simulink model "c00005M_harness"  (R2018a)
settings: Solver=FixedStepAuto  StartTime=0.0  StopTime=300  FixedStep=0.1  RelTol=1e-3
undefined symbols (not defined in the file): A1, hmax, PriorityTank, R1, R2, sigbuilder_block, TempThreshold
(part 5 of 50)

== system c00005M_harness/M007 ==
  note: VALUES
      | ---------------------------------
      | ControlType = 1 | 2 | 3
      | FillTank = 0 | 1
      | EmptyTank = 0 | 1
      | ManualReference between 0 and 1
      | Tempreature between 0 and 100
      | EmergencyButton = 0 | 1
      | LiquidLevel between 0 and 1 (hmax)
  note: Inputs For Tank2
  note: NAMES
      | --------------------------------------------
      | CT1 = ControlType Tank 1
      | F1 = Fill Tank 1
      | E1 = Empty Tank 1
      | MR1 = Manual Reference Tank1
      | T1 = Temperature Tank 1
      | EB1 = Emergency Button Tank 1
      | LL1 = Liquid Level 1
  note: Inputs For Tank3
  note: Inputs For Tank1
  CT1 : Inport
  F1 : Inport  Port=2
  E1 : Inport  Port=3
  T1 : Inport  Port=4
  EB1 : Inport  Port=5
  CT3 : Inport  Port=6
  F3 : Inport  Port=7
  E3 : Inport  Port=8
  T3 : Inport  Port=9
  EB3 : Inport  Port=10
  Tank1 : Subsystem
  Tank3 : Subsystem
  LL1 : Outport
  LL3 : Outport  Port=2
  wires:
  EB1/1 -> Tank1/5(EB1)
  Tank3/1(LL3) -> LL3/1, Tank1/6(LL3)
  T1/1 -> Tank1/4(T1)
  Tank1/1(LL1) -> LL1/1, Tank3/6(LL1)
  E3/1 -> Tank3/3(E3)
  F1/1 -> Tank1/2(F1)
  E1/1 -> Tank1/3(E1)
  CT3/1 -> Tank3/1(CT3)
  F3/1 -> Tank3/2(F3)
  EB3/1 -> Tank3/5(EB3)
  T3/1 -> Tank3/4(T3)
  CT1/1 -> Tank1/1(CT1)

== system c00005M_harness/M008 ==
  note: VALUES
      | ---------------------------------
      | ControlType = 1 | 2 | 3
      | FillTank = 0 | 1
      | EmptyTank = 0 | 1
      | ManualReference between 0 and 1
      | Tempreature between 0 and 100
      | EmergencyButton = 0 | 1
      | LiquidLevel between 0 and 1 (hmax)
  note: Inputs For Tank2
  note: NAMES
      | --------------------------------------------
      | CT1 = ControlType Tank 1
      | F1 = Fill Tank 1
      | E1 = Empty Tank 1
      | MR1 = Manual Reference Tank1
      | T1 = Temperature Tank 1
      | EB1 = Emergency Button Tank 1
      | LL1 = Liquid Level 1
  note: Inputs For Tank3
  note: Inputs For Tank1
  CT1 : Inport
  F1 : Inport  Port=2
  E1 : Inport  Port=3
  T1 : Inport  Port=4
  EB1 : Inport  Port=5
  CT3 : Inport  Port=6
  F3 : Inport  Port=7
  E3 : Inport  Port=8
  T3 : Inport  Port=9
  EB3 : Inport  Port=10
  Tank1 : Subsystem
  Tank3 : Subsystem
  LL1 : Outport
  LL3 : Outport  Port=2
  wires:
  EB1/1 -> Tank1/5(EB1)
  Tank3/1(LL3) -> LL3/1, Tank1/6(LL3)
  T1/1 -> Tank1/4(T1)
  Tank1/1(LL1) -> LL1/1, Tank3/6(LL1)
  E3/1 -> Tank3/3(E3)
  F1/1 -> Tank1/2(F1)
  E1/1 -> Tank1/3(E1)
  CT3/1 -> Tank3/1(CT3)
  F3/1 -> Tank3/2(F3)
  EB3/1 -> Tank3/5(EB3)
  T3/1 -> Tank3/4(T3)
  CT1/1 -> Tank1/1(CT1)

== system c00005M_harness/M009 ==
  note: VALUES
      | ---------------------------------
      | ControlType = 1 | 2 | 3
      | FillTank = 0 | 1
      | EmptyTank = 0 | 1
      | ManualReference between 0 and 1
      | Tempreature between 0 and 100
      | EmergencyButton = 0 | 1
      | LiquidLevel between 0 and 1 (hmax)
  note: Inputs For Tank2
  note: NAMES
      | --------------------------------------------
      | CT1 = ControlType Tank 1
      | F1 = Fill Tank 1
      | E1 = Empty Tank 1
      | MR1 = Manual Reference Tank1
      | T1 = Temperature Tank 1
      | EB1 = Emergency Button Tank 1
      | LL1 = Liquid Level 1
  note: Inputs For Tank3
  note: Inputs For Tank1
  CT1 : Inport
  F1 : Inport  Port=2
  E1 : Inport  Port=3
  T1 : Inport  Port=4
  EB1 : Inport  Port=5
  CT3 : Inport  Port=6
  F3 : Inport  Port=7
  E3 : Inport  Port=8
  T3 : Inport  Port=9
  EB3 : Inport  Port=10
  Tank1 : Subsystem
  Tank3 : Subsystem
  LL1 : Outport
  LL3 : Outport  Port=2
  wires:
  EB1/1 -> Tank1/5(EB1)
  Tank3/1(LL3) -> LL3/1, Tank1/6(LL3)
  T1/1 -> Tank1/4(T1)
  Tank1/1(LL1) -> LL1/1, Tank3/6(LL1)
  E3/1 -> Tank3/3(E3)
  F1/1 -> Tank1/2(F1)
  E1/1 -> Tank1/3(E1)
  CT3/1 -> Tank3/1(CT3)
  F3/1 -> Tank3/2(F3)
  EB3/1 -> Tank3/5(EB3)
  T3/1 -> Tank3/4(T3)
  CT1/1 -> Tank1/1(CT1)

== system c00005M_harness/M010 ==
  note: VALUES
      | ---------------------------------
      | ControlType = 1 | 2 | 3
      | FillTank = 0 | 1
      | EmptyTank = 0 | 1
      | ManualReference between 0 and 1
      | Tempreature between 0 and 100
      | EmergencyButton = 0 | 1
      | LiquidLevel between 0 and 1 (hmax)
  note: Inputs For Tank2
  note: NAMES
      | --------------------------------------------
      | CT1 = ControlType Tank 1
      | F1 = Fill Tank 1
      | E1 = Empty Tank 1
      | MR1 = Manual Reference Tank1
      | T1 = Temperature Tank 1
      | EB1 = Emergency Button Tank 1
      | LL1 = Liquid Level 1
  note: Inputs For Tank3
  note: Inputs For Tank1
  CT1 : Inport
  F1 : Inport  Port=2
  E1 : Inport  Port=3
  T1 : Inport  Port=4
  EB1 : Inport  Port=5
  CT3 : Inport  Port=6
  F3 : Inport  Port=7
  E3 : Inport  Port=8
  T3 : Inport  Port=9
  EB3 : Inport  Port=10
  Tank1 : Subsystem
  Tank3 : Subsystem
  LL1 : Outport
  LL3 : Outport  Port=2
  wires:
  EB1/1 -> Tank1/5(EB1)
  Tank3/1(LL3) -> LL3/1, Tank1/6(LL3)
  T1/1 -> Tank1/4(T1)
  Tank1/1(LL1) -> LL1/1, Tank3/6(LL1)
  E3/1 -> Tank3/3(E3)
  F1/1 -> Tank1/2(F1)
  E1/1 -> Tank1/3(E1)
  CT3/1 -> Tank3/1(CT3)
  F3/1 -> Tank3/2(F3)
  EB3/1 -> Tank3/5(EB3)
  T3/1 -> Tank3/4(T3)
  CT1/1 -> Tank1/1(CT1)

== system c00005M_harness/M011 ==
  note: VALUES
      | ---------------------------------
      | ControlType = 1 | 2 | 3
      | FillTank = 0 | 1
      | EmptyTank = 0 | 1
      | ManualReference between 0 and 1
      | Tempreature between 0 and 100
      | EmergencyButton = 0 | 1
      | LiquidLevel between 0 and 1 (hmax)
  note: Inputs For Tank2
  note: NAMES
      | --------------------------------------------
      | CT1 = ControlType Tank 1
      | F1 = Fill Tank 1
      | E1 = Empty Tank 1
      | MR1 = Manual Reference Tank1
      | T1 = Temperature Tank 1
      | EB1 = Emergency Button Tank 1
      | LL1 = Liquid Level 1
  note: Inputs For Tank3
  note: Inputs For Tank1
  CT1 : Inport
  F1 : Inport  Port=2
  E1 : Inport  Port=3
  T1 : Inport  Port=4
  EB1 : Inport  Port=5
  CT3 : Inport  Port=6
  F3 : Inport  Port=7
  E3 : Inport  Port=8
  T3 : Inport  Port=9
  EB3 : Inport  Port=10
  Tank1 : Subsystem
  Tank3 : Subsystem
  LL1 : Outport
  LL3 : Outport  Port=2
  wires:
  EB1/1 -> Tank1/5(EB1)
  Tank3/1(LL3) -> LL3/1, Tank1/6(LL3)
  T1/1 -> Tank1/4(T1)
  Tank1/1(LL1) -> LL1/1, Tank3/6(LL1)
  E3/1 -> Tank3/3(E3)
  F1/1 -> Tank1/2(F1)
  E1/1 -> Tank1/3(E1)
  CT3/1 -> Tank3/1(CT3)
  F3/1 -> Tank3/2(F3)
  EB3/1 -> Tank3/5(EB3)
  T3/1 -> Tank3/4(T3)
  CT1/1 -> Tank1/1(CT1)

== system c00005M_harness/M012 ==
  note: VALUES
      | ---------------------------------
      | ControlType = 1 | 2 | 3
      | FillTank = 0 | 1
      | EmptyTank = 0 | 1
      | ManualReference between 0 and 1
      | Tempreature between 0 and 100
      | EmergencyButton = 0 | 1
      | LiquidLevel between 0 and 1 (hmax)
  note: Inputs For Tank2
  note: NAMES
      | --------------------------------------------
      | CT1 = ControlType Tank 1
      | F1 = Fill Tank 1
      | E1 = Empty Tank 1
      | MR1 = Manual Reference Tank1
      | T1 = Temperature Tank 1
      | EB1 = Emergency Button Tank 1
      | LL1 = Liquid Level 1
  note: Inputs For Tank3
  note: Inputs For Tank1
  CT1 : Inport
  F1 : Inport  Port=2
  E1 : Inport  Port=3
  T1 : Inport  Port=4
  EB1 : Inport  Port=5
  CT3 : Inport  Port=6
  F3 : Inport  Port=7
  E3 : Inport  Port=8
  T3 : Inport  Port=9
  EB3 : Inport  Port=10
  Tank1 : Subsystem
  Tank3 : Subsystem
  LL1 : Outport
  LL3 : Outport  Port=2
  wires:
  EB1/1 -> Tank1/5(EB1)
  Tank3/1(LL3) -> LL3/1, Tank1/6(LL3)
  T1/1 -> Tank1/4(T1)
  Tank1/1(LL1) -> LL1/1, Tank3/6(LL1)
  E3/1 -> Tank3/3(E3)
  F1/1 -> Tank1/2(F1)
  E1/1 -> Tank1/3(E1)
  CT3/1 -> Tank3/1(CT3)
  F3/1 -> Tank3/2(F3)
  EB3/1 -> Tank3/5(EB3)
  T3/1 -> Tank3/4(T3)
  CT1/1 -> Tank1/1(CT1)

== system c00005M_harness/M013 ==
  note: VALUES
      | ---------------------------------
      | ControlType = 1 | 2 | 3
      | FillTank = 0 | 1
      | EmptyTank = 0 | 1
      | ManualReference between 0 and 1
      | Tempreature between 0 and 100
      | EmergencyButton = 0 | 1
      | LiquidLevel between 0 and 1 (hmax)
  note: Inputs For Tank2
  note: NAMES
      | --------------------------------------------
      | CT1 = ControlType Tank 1
      | F1 = Fill Tank 1
      | E1 = Empty Tank 1
      | MR1 = Manual Reference Tank1
      | T1 = Temperature Tank 1
      | EB1 = Emergency Button Tank 1
      | LL1 = Liquid Level 1
  note: Inputs For Tank3
  note: Inputs For Tank1
  CT1 : Inport
  F1 : Inport  Port=2
  E1 : Inport  Port=3
  T1 : Inport  Port=4
  EB1 : Inport  Port=5
  CT3 : Inport  Port=6
  F3 : Inport  Port=7
  E3 : Inport  Port=8
  T3 : Inport  Port=9
  EB3 : Inport  Port=10
  Tank1 : Subsystem
  Tank3 : Subsystem
  LL1 : Outport
  LL3 : Outport  Port=2
  wires:
  EB1/1 -> Tank1/5(EB1)
  Tank3/1(LL3) -> LL3/1, Tank1/6(LL3)
  T1/1 -> Tank1/4(T1)
  Tank1/1(LL1) -> LL1/1, Tank3/6(LL1)
  E3/1 -> Tank3/3(E3)
  F1/1 -> Tank1/2(F1)
  E1/1 -> Tank1/3(E1)
  CT3/1 -> Tank3/1(CT3)
  F3/1 -> Tank3/2(F3)
  EB3/1 -> Tank3/5(EB3)
  T3/1 -> Tank3/4(T3)
  CT1/1 -> Tank1/1(CT1)

== system c00005M_harness/M014 ==
  note: VALUES
      | ---------------------------------
      | ControlType = 1 | 2 | 3
      | FillTank = 0 | 1
      | EmptyTank = 0 | 1
      | ManualReference between 0 and 1
      | Tempreature between 0 and 100
      | EmergencyButton = 0 | 1
      | LiquidLevel between 0 and 1 (hmax)
  note: Inputs For Tank2
  note: NAMES
      | --------------------------------------------
      | CT1 = ControlType Tank 1
      | F1 = Fill Tank 1
      | E1 = Empty Tank 1
      | MR1 = Manual Reference Tank1
      | T1 = Temperature Tank 1
      | EB1 = Emergency Button Tank 1
      | LL1 = Liquid Level 1
  note: Inputs For Tank3
  note: Inputs For Tank1
  CT1 : Inport
  F1 : Inport  Port=2
  E1 : Inport  Port=3
  T1 : Inport  Port=4
  EB1 : Inport  Port=5
  CT3 : Inport  Port=6
  F3 : Inport  Port=7
  E3 : Inport  Port=8
  T3 : Inport  Port=9
  EB3 : Inport  Port=10
  Tank1 : Subsystem
  Tank3 : Subsystem
  LL1 : Outport
  LL3 : Outport  Port=2
  wires:
  EB1/1 -> Tank1/5(EB1)
  Tank3/1(LL3) -> LL3/1, Tank1/6(LL3)
  T1/1 -> Tank1/4(T1)
  Tank1/1(LL1) -> LL1/1, Tank3/6(LL1)
  E3/1 -> Tank3/3(E3)
  F1/1 -> Tank1/2(F1)
  E1/1 -> Tank1/3(E1)
  CT3/1 -> Tank3/1(CT3)
  F3/1 -> Tank3/2(F3)
  EB3/1 -> Tank3/5(EB3)
  T3/1 -> Tank3/4(T3)
  CT1/1 -> Tank1/1(CT1)

== system c00005M_harness/M015 ==
  note: VALUES
      | ---------------------------------
      | ControlType = 1 | 2 | 3
      | FillTank = 0 | 1
      | EmptyTank = 0 | 1
      | ManualReference between 0 and 1
      | Tempreature between 0 and 100
      | EmergencyButton = 0 | 1
      | LiquidLevel between 0 and 1 (hmax)
  note: Inputs For Tank2
  note: NAMES
      | --------------------------------------------
      | CT1 = ControlType Tank 1
      | F1 = Fill Tank 1
      | E1 = Empty Tank 1
      | MR1 = Manual Reference Tank1
      | T1 = Temperature Tank 1
      | EB1 = Emergency Button Tank 1
      | LL1 = Liquid Level 1
  note: Inputs For Tank3
  note: Inputs For Tank1
  CT1 : Inport
  F1 : Inport  Port=2
  E1 : Inport  Port=3
  T1 : Inport  Port=4
  EB1 : Inport  Port=5
  CT3 : Inport  Port=6
  F3 : Inport  Port=7
  E3 : Inport  Port=8
  T3 : Inport  Port=9
  EB3 : Inport  Port=10
  Tank1 : Subsystem
  Tank3 : Subsystem
  LL1 : Outport
  LL3 : Outport  Port=2
  wires:
  EB1/1 -> Tank1/5(EB1)
  Tank3/1(LL3) -> LL3/1, Tank1/6(LL3)
  T1/1 -> Tank1/4(T1)
  Tank1/1(LL1) -> LL1/1, Tank3/6(LL1)
  E3/1 -> Tank3/3(E3)
  F1/1 -> Tank1/2(F1)
  E1/1 -> Tank1/3(E1)
  CT3/1 -> Tank3/1(CT3)
  F3/1 -> Tank3/2(F3)
  EB3/1 -> Tank3/5(EB3)
  T3/1 -> Tank3/4(T3)
  CT1/1 -> Tank1/1(CT1)

== system c00005M_harness/M016 ==
  note: VALUES
      | ---------------------------------
      | ControlType = 1 | 2 | 3
      | FillTank = 0 | 1
      | EmptyTank = 0 | 1
      | ManualReference between 0 and 1
      | Tempreature between 0 and 100
      | EmergencyButton = 0 | 1
      | LiquidLevel between 0 and 1 (hmax)
  note: Inputs For Tank2
  note: NAMES
      | --------------------------------------------
      | CT1 = ControlType Tank 1
      | F1 = Fill Tank 1
      | E1 = Empty Tank 1
      | MR1 = Manual Reference Tank1
      | T1 = Temperature Tank 1
      | EB1 = Emergency Button Tank 1
      | LL1 = Liquid Level 1
  note: Inputs For Tank3
  note: Inputs For Tank1
  CT1 : Inport
  F1 : Inport  Port=2
  E1 : Inport  Port=3
  T1 : Inport  Port=4
  EB1 : Inport  Port=5
  CT3 : Inport  Port=6
  F3 : Inport  Port=7
  E3 : Inport  Port=8
  T3 : Inport  Port=9
  EB3 : Inport  Port=10
  Tank1 : Subsystem
  Tank3 : Subsystem
  LL1 : Outport
  LL3 : Outport  Port=2
  wires:
  EB1/1 -> Tank1/5(EB1)
  Tank3/1(LL3) -> LL3/1, Tank1/6(LL3)
  T1/1 -> Tank1/4(T1)
  Tank1/1(LL1) -> LL1/1, Tank3/6(LL1)
  E3/1 -> Tank3/3(E3)
  F1/1 -> Tank1/2(F1)
  E1/1 -> Tank1/3(E1)
  CT3/1 -> Tank3/1(CT3)
  F3/1 -> Tank3/2(F3)
  EB3/1 -> Tank3/5(EB3)
  T3/1 -> Tank3/4(T3)
  CT1/1 -> Tank1/1(CT1)

== system c00005M_harness/M017 ==
  note: VALUES
      | ---------------------------------
      | ControlType = 1 | 2 | 3
      | FillTank = 0 | 1
      | EmptyTank = 0 | 1
      | ManualReference between 0 and 1
      | Tempreature between 0 and 100
      | EmergencyButton = 0 | 1
      | LiquidLevel between 0 and 1 (hmax)
  note: Inputs For Tank2
  note: NAMES
      | --------------------------------------------
      | CT1 = ControlType Tank 1
      | F1 = Fill Tank 1
      | E1 = Empty Tank 1
      | MR1 = Manual Reference Tank1
      | T1 = Temperature Tank 1
      | EB1 = Emergency Button Tank 1
      | LL1 = Liquid Level 1
  note: Inputs For Tank3
  note: Inputs For Tank1
  CT1 : Inport
  F1 : Inport  Port=2
  E1 : Inport  Port=3
  T1 : Inport  Port=4
  EB1 : Inport  Port=5
  CT3 : Inport  Port=6
  F3 : Inport  Port=7
  E3 : Inport  Port=8
  T3 : Inport  Port=9
  EB3 : Inport  Port=10
  Tank1 : Subsystem
  Tank3 : Subsystem
  LL1 : Outport
  LL3 : Outport  Port=2
  wires:
  EB1/1 -> Tank1/5(EB1)
  Tank3/1(LL3) -> LL3/1, Tank1/6(LL3)
  T1/1 -> Tank1/4(T1)
  Tank1/1(LL1) -> LL1/1, Tank3/6(LL1)
  E3/1 -> Tank3/3(E3)
  F1/1 -> Tank1/2(F1)
  E1/1 -> Tank1/3(E1)
  CT3/1 -> Tank3/1(CT3)
  F3/1 -> Tank3/2(F3)
  EB3/1 -> Tank3/5(EB3)
  T3/1 -> Tank3/4(T3)
  CT1/1 -> Tank1/1(CT1)

== system c00005M_harness/M018 ==
  note: VALUES
      | ---------------------------------
      | ControlType = 1 | 2 | 3
      | FillTank = 0 | 1
      | EmptyTank = 0 | 1
      | ManualReference between 0 and 1
      | Tempreature between 0 and 100
      | EmergencyButton = 0 | 1
      | LiquidLevel between 0 and 1 (hmax)
  note: Inputs For Tank2
  note: NAMES
      | --------------------------------------------
      | CT1 = ControlType Tank 1
      | F1 = Fill Tank 1
      | E1 = Empty Tank 1
      | MR1 = Manual Reference Tank1
      | T1 = Temperature Tank 1
      | EB1 = Emergency Button Tank 1
      | LL1 = Liquid Level 1
  note: Inputs For Tank3
  note: Inputs For Tank1
  CT1 : Inport
  F1 : Inport  Port=2
  E1 : Inport  Port=3
  T1 : Inport  Port=4
  EB1 : Inport  Port=5
  CT3 : Inport  Port=6
  F3 : Inport  Port=7
  E3 : Inport  Port=8
  T3 : Inport  Port=9
  EB3 : Inport  Port=10
  Tank1 : Subsystem
  Tank3 : Subsystem
  LL1 : Outport
  LL3 : Outport  Port=2
  wires:
  EB1/1 -> Tank1/5(EB1)
  Tank3/1(LL3) -> LL3/1, Tank1/6(LL3)
  T1/1 -> Tank1/4(T1)
  Tank1/1(LL1) -> LL1/1, Tank3/6(LL1)
  E3/1 -> Tank3/3(E3)
  F1/1 -> Tank1/2(F1)
  E1/1 -> Tank1/3(E1)
  CT3/1 -> Tank3/1(CT3)
  F3/1 -> Tank3/2(F3)
  EB3/1 -> Tank3/5(EB3)
  T3/1 -> Tank3/4(T3)
  CT1/1 -> Tank1/1(CT1)

== system c00005M_harness/M019 ==
  note: VALUES
      | ---------------------------------
      | ControlType = 1 | 2 | 3
      | FillTank = 0 | 1
      | EmptyTank = 0 | 1
      | ManualReference between 0 and 1
      | Tempreature between 0 and 100
      | EmergencyButton = 0 | 1
      | LiquidLevel between 0 and 1 (hmax)
  note: Inputs For Tank2
  note: NAMES
      | --------------------------------------------
      | CT1 = ControlType Tank 1
      | F1 = Fill Tank 1
      | E1 = Empty Tank 1
      | MR1 = Manual Reference Tank1
      | T1 = Temperature Tank 1
      | EB1 = Emergency Button Tank 1
      | LL1 = Liquid Level 1
  note: Inputs For Tank3
  note: Inputs For Tank1
  CT1 : Inport
  F1 : Inport  Port=2
  E1 : Inport  Port=3
  T1 : Inport  Port=4
  EB1 : Inport  Port=5
  CT3 : Inport  Port=6
  F3 : Inport  Port=7
  E3 : Inport  Port=8
  T3 : Inport  Port=9
  EB3 : Inport  Port=10
  Tank1 : Subsystem
  Tank3 : Subsystem
  LL1 : Outport
  LL3 : Outport  Port=2
  wires:
  EB1/1 -> Tank1/5(EB1)
  Tank3/1(LL3) -> LL3/1, Tank1/6(LL3)
  T1/1 -> Tank1/4(T1)
  Tank1/1(LL1) -> LL1/1, Tank3/6(LL1)
  E3/1 -> Tank3/3(E3)
  F1/1 -> Tank1/2(F1)
  E1/1 -> Tank1/3(E1)
  CT3/1 -> Tank3/1(CT3)
  F3/1 -> Tank3/2(F3)
  EB3/1 -> Tank3/5(EB3)
  T3/1 -> Tank3/4(T3)
  CT1/1 -> Tank1/1(CT1)

== system c00005M_harness/M020 ==
  note: VALUES
      | ---------------------------------
      | ControlType = 1 | 2 | 3
      | FillTank = 0 | 1
      | EmptyTank = 0 | 1
      | ManualReference between 0 and 1
      | Tempreature between 0 and 100
      | EmergencyButton = 0 | 1
      | LiquidLevel between 0 and 1 (hmax)
  note: Inputs For Tank2
  note: NAMES
      | --------------------------------------------
      | CT1 = ControlType Tank 1
      | F1 = Fill Tank 1
      | E1 = Empty Tank 1
      | MR1 = Manual Reference Tank1
      | T1 = Temperature Tank 1
      | EB1 = Emergency Button Tank 1
      | LL1 = Liquid Level 1
  note: Inputs For Tank3
  note: Inputs For Tank1
  CT1 : Inport
  F1 : Inport  Port=2
  E1 : Inport  Port=3
  T1 : Inport  Port=4
  EB1 : Inport  Port=5
  CT3 : Inport  Port=6
  F3 : Inport  Port=7
  E3 : Inport  Port=8
  T3 : Inport  Port=9
  EB3 : Inport  Port=10
  Tank1 : Subsystem
  Tank3 : Subsystem
  LL1 : Outport
  LL3 : Outport  Port=2
  wires:
  EB1/1 -> Tank1/5(EB1)
  Tank3/1(LL3) -> LL3/1, Tank1/6(LL3)
  T1/1 -> Tank1/4(T1)
  Tank1/1(LL1) -> LL1/1, Tank3/6(LL1)
  E3/1 -> Tank3/3(E3)
  F1/1 -> Tank1/2(F1)
  E1/1 -> Tank1/3(E1)
  CT3/1 -> Tank3/1(CT3)
  F3/1 -> Tank3/2(F3)
  EB3/1 -> Tank3/5(EB3)
  T3/1 -> Tank3/4(T3)
  CT1/1 -> Tank1/1(CT1)

== system c00005M_harness/M021 ==
  note: VALUES
      | ---------------------------------
      | ControlType = 1 | 2 | 3
      | FillTank = 0 | 1
      | EmptyTank = 0 | 1
      | ManualReference between 0 and 1
      | Tempreature between 0 and 100
      | EmergencyButton = 0 | 1
      | LiquidLevel between 0 and 1 (hmax)
  note: Inputs For Tank2
  note: NAMES
      | --------------------------------------------
      | CT1 = ControlType Tank 1
      | F1 = Fill Tank 1
      | E1 = Empty Tank 1
      | MR1 = Manual Reference Tank1
      | T1 = Temperature Tank 1
      | EB1 = Emergency Button Tank 1
      | LL1 = Liquid Level 1
  note: Inputs For Tank3
  note: Inputs For Tank1
  CT1 : Inport
  F1 : Inport  Port=2
  E1 : Inport  Port=3
  T1 : Inport  Port=4
  EB1 : Inport  Port=5
  CT3 : Inport  Port=6
  F3 : Inport  Port=7
  E3 : Inport  Port=8
  T3 : Inport  Port=9
  EB3 : Inport  Port=10
  Tank1 : Subsystem
  Tank3 : Subsystem
  LL1 : Outport
  LL3 : Outport  Port=2
  wires:
  EB1/1 -> Tank1/5(EB1)
  Tank3/1(LL3) -> LL3/1, Tank1/6(LL3)
  T1/1 -> Tank1/4(T1)
  Tank1/1(LL1) -> LL1/1, Tank3/6(LL1)
  E3/1 -> Tank3/3(E3)
  F1/1 -> Tank1/2(F1)
  E1/1 -> Tank1/3(E1)
  CT3/1 -> Tank3/1(CT3)
  F3/1 -> Tank3/2(F3)
  EB3/1 -> Tank3/5(EB3)
  T3/1 -> Tank3/4(T3)
  CT1/1 -> Tank1/1(CT1)

== system c00005M_harness/M022 ==
  note: VALUES
      | ---------------------------------
      | ControlType = 1 | 2 | 3
      | FillTank = 0 | 1
      | EmptyTank = 0 | 1
      | ManualReference between 0 and 1
      | Tempreature between 0 and 100
      | EmergencyButton = 0 | 1
      | LiquidLevel between 0 and 1 (hmax)
  note: Inputs For Tank2
  note: NAMES
      | --------------------------------------------
      | CT1 = ControlType Tank 1
      | F1 = Fill Tank 1
      | E1 = Empty Tank 1
      | MR1 = Manual Reference Tank1
      | T1 = Temperature Tank 1
      | EB1 = Emergency Button Tank 1
      | LL1 = Liquid Level 1
  note: Inputs For Tank3
  note: Inputs For Tank1
  CT1 : Inport
  F1 : Inport  Port=2
  E1 : Inport  Port=3
  T1 : Inport  Port=4
  EB1 : Inport  Port=5
  CT3 : Inport  Port=6
  F3 : Inport  Port=7
  E3 : Inport  Port=8
  T3 : Inport  Port=9
  EB3 : Inport  Port=10
  Tank1 : Subsystem
  Tank3 : Subsystem
  LL1 : Outport
  LL3 : Outport  Port=2
  wires:
  EB1/1 -> Tank1/5(EB1)
  Tank3/1(LL3) -> LL3/1, Tank1/6(LL3)
  T1/1 -> Tank1/4(T1)
  Tank1/1(LL1) -> LL1/1, Tank3/6(LL1)
  E3/1 -> Tank3/3(E3)
  F1/1 -> Tank1/2(F1)
  E1/1 -> Tank1/3(E1)
  CT3/1 -> Tank3/1(CT3)
  F3/1 -> Tank3/2(F3)
  EB3/1 -> Tank3/5(EB3)
  T3/1 -> Tank3/4(T3)
  CT1/1 -> Tank1/1(CT1)

== system c00005M_harness/M023 ==
  note: VALUES
      | ---------------------------------
      | ControlType = 1 | 2 | 3
      | FillTank = 0 | 1
      | EmptyTank = 0 | 1
      | ManualReference between 0 and 1
      | Tempreature between 0 and 100
      | EmergencyButton = 0 | 1
      | LiquidLevel between 0 and 1 (hmax)
  note: Inputs For Tank2
  note: NAMES
      | --------------------------------------------
      | CT1 = ControlType Tank 1
      | F1 = Fill Tank 1
      | E1 = Empty Tank 1
      | MR1 = Manual Reference Tank1
      | T1 = Temperature Tank 1
      | EB1 = Emergency Button Tank 1
      | LL1 = Liquid Level 1
  note: Inputs For Tank3
  note: Inputs For Tank1
  CT1 : Inport
  F1 : Inport  Port=2
  E1 : Inport  Port=3
  T1 : Inport  Port=4
  EB1 : Inport  Port=5
  CT3 : Inport  Port=6
  F3 : Inport  Port=7
  E3 : Inport  Port=8
  T3 : Inport  Port=9
  EB3 : Inport  Port=10
  Tank1 : Subsystem
  Tank3 : Subsystem
  LL1 : Outport
  LL3 : Outport  Port=2
  wires:
  EB1/1 -> Tank1/5(EB1)
  Tank3/1(LL3) -> LL3/1, Tank1/6(LL3)
  T1/1 -> Tank1/4(T1)
  Tank1/1(LL1) -> LL1/1, Tank3/6(LL1)
  E3/1 -> Tank3/3(E3)
  F1/1 -> Tank1/2(F1)
  E1/1 -> Tank1/3(E1)
  CT3/1 -> Tank3/1(CT3)
  F3/1 -> Tank3/2(F3)
  EB3/1 -> Tank3/5(EB3)
  T3/1 -> Tank3/4(T3)
  CT1/1 -> Tank1/1(CT1)

== system c00005M_harness/M024 ==
  note: VALUES
      | ---------------------------------
      | ControlType = 1 | 2 | 3
      | FillTank = 0 | 1
      | EmptyTank = 0 | 1
      | ManualReference between 0 and 1
      | Tempreature between 0 and 100
      | EmergencyButton = 0 | 1
      | LiquidLevel between 0 and 1 (hmax)
  note: Inputs For Tank2
  note: NAMES
      | --------------------------------------------
      | CT1 = ControlType Tank 1
      | F1 = Fill Tank 1
      | E1 = Empty Tank 1
      | MR1 = Manual Reference Tank1
      | T1 = Temperature Tank 1
      | EB1 = Emergency Button Tank 1
      | LL1 = Liquid Level 1
  note: Inputs For Tank3
  note: Inputs For Tank1
  CT1 : Inport
  F1 : Inport  Port=2
  E1 : Inport  Port=3
  T1 : Inport  Port=4
  EB1 : Inport  Port=5
  CT3 : Inport  Port=6
  F3 : Inport  Port=7
  E3 : Inport  Port=8
  T3 : Inport  Port=9
  EB3 : Inport  Port=10
  Tank1 : Subsystem
  Tank3 : Subsystem
  LL1 : Outport
  LL3 : Outport  Port=2
  wires:
  EB1/1 -> Tank1/5(EB1)
  Tank3/1(LL3) -> LL3/1, Tank1/6(LL3)
  T1/1 -> Tank1/4(T1)
  Tank1/1(LL1) -> LL1/1, Tank3/6(LL1)
  E3/1 -> Tank3/3(E3)
  F1/1 -> Tank1/2(F1)
  E1/1 -> Tank1/3(E1)
  CT3/1 -> Tank3/1(CT3)
  F3/1 -> Tank3/2(F3)
  EB3/1 -> Tank3/5(EB3)
  T3/1 -> Tank3/4(T3)
  CT1/1 -> Tank1/1(CT1)

== system c00005M_harness/M025 ==
  note: VALUES
      | ---------------------------------
      | ControlType = 1 | 2 | 3
      | FillTank = 0 | 1
      | EmptyTank = 0 | 1
      | ManualReference between 0 and 1
      | Tempreature between 0 and 100
      | EmergencyButton = 0 | 1
      | LiquidLevel between 0 and 1 (hmax)
  note: Inputs For Tank2
  note: NAMES
      | --------------------------------------------
      | CT1 = ControlType Tank 1
      | F1 = Fill Tank 1
      | E1 = Empty Tank 1
      | MR1 = Manual Reference Tank1
      | T1 = Temperature Tank 1
      | EB1 = Emergency Button Tank 1
      | LL1 = Liquid Level 1
  note: Inputs For Tank3
  note: Inputs For Tank1
  CT1 : Inport
  F1 : Inport  Port=2
  E1 : Inport  Port=3
  T1 : Inport  Port=4
  EB1 : Inport  Port=5
  CT3 : Inport  Port=6
  F3 : Inport  Port=7
  E3 : Inport  Port=8
  T3 : Inport  Port=9
  EB3 : Inport  Port=10
  Tank1 : Subsystem
  Tank3 : Subsystem
  LL1 : Outport
  LL3 : Outport  Port=2
  wires:
  EB1/1 -> Tank1/5(EB1)
  Tank3/1(LL3) -> LL3/1, Tank1/6(LL3)
  T1/1 -> Tank1/4(T1)
  Tank1/1(LL1) -> LL1/1, Tank3/6(LL1)
  E3/1 -> Tank3/3(E3)
  F1/1 -> Tank1/2(F1)
  E1/1 -> Tank1/3(E1)
  CT3/1 -> Tank3/1(CT3)
  F3/1 -> Tank3/2(F3)
  EB3/1 -> Tank3/5(EB3)
  T3/1 -> Tank3/4(T3)
  CT1/1 -> Tank1/1(CT1)

== system c00005M_harness/M026 ==
  note: VALUES
      | ---------------------------------
      | ControlType = 1 | 2 | 3
      | FillTank = 0 | 1
      | EmptyTank = 0 | 1
      | ManualReference between 0 and 1
      | Tempreature between 0 and 100
      | EmergencyButton = 0 | 1
      | LiquidLevel between 0 and 1 (hmax)
  note: Inputs For Tank2
  note: NAMES
      | --------------------------------------------
      | CT1 = ControlType Tank 1
      | F1 = Fill Tank 1
      | E1 = Empty Tank 1
      | MR1 = Manual Reference Tank1
      | T1 = Temperature Tank 1
      | EB1 = Emergency Button Tank 1
      | LL1 = Liquid Level 1
  note: Inputs For Tank3
  note: Inputs For Tank1
  CT1 : Inport
  F1 : Inport  Port=2
  E1 : Inport  Port=3
  T1 : Inport  Port=4
  EB1 : Inport  Port=5
  CT3 : Inport  Port=6
  F3 : Inport  Port=7
  E3 : Inport  Port=8
  T3 : Inport  Port=9
  EB3 : Inport  Port=10
  Tank1 : Subsystem
  Tank3 : Subsystem
  LL1 : Outport
  LL3 : Outport  Port=2
  wires:
  EB1/1 -> Tank1/5(EB1)
  Tank3/1(LL3) -> LL3/1, Tank1/6(LL3)
  T1/1 -> Tank1/4(T1)
  Tank1/1(LL1) -> LL1/1, Tank3/6(LL1)
  E3/1 -> Tank3/3(E3)
  F1/1 -> Tank1/2(F1)
  E1/1 -> Tank1/3(E1)
  CT3/1 -> Tank3/1(CT3)
  F3/1 -> Tank3/2(F3)
  EB3/1 -> Tank3/5(EB3)
  T3/1 -> Tank3/4(T3)
  CT1/1 -> Tank1/1(CT1)

== system c00005M_harness/M027 ==
  note: VALUES
      | ---------------------------------
      | ControlType = 1 | 2 | 3
      | FillTank = 0 | 1
      | EmptyTank = 0 | 1
      | ManualReference between 0 and 1
      | Tempreature between 0 and 100
      | EmergencyButton = 0 | 1
      | LiquidLevel between 0 and 1 (hmax)
  note: Inputs For Tank2
  note: NAMES
      | --------------------------------------------
      | CT1 = ControlType Tank 1
      | F1 = Fill Tank 1
      | E1 = Empty Tank 1
      | MR1 = Manual Reference Tank1
      | T1 = Temperature Tank 1
      | EB1 = Emergency Button Tank 1
      | LL1 = Liquid Level 1
  note: Inputs For Tank3
  note: Inputs For Tank1
  CT1 : Inport
  F1 : Inport  Port=2
  E1 : Inport  Port=3
  T1 : Inport  Port=4
  EB1 : Inport  Port=5
  CT3 : Inport  Port=6
  F3 : Inport  Port=7
  E3 : Inport  Port=8
  T3 : Inport  Port=9
  EB3 : Inport  Port=10
  Tank1 : Subsystem
  Tank3 : Subsystem
  LL1 : Outport
  LL3 : Outport  Port=2
  wires:
  EB1/1 -> Tank1/5(EB1)
  Tank3/1(LL3) -> LL3/1, Tank1/6(LL3)
  T1/1 -> Tank1/4(T1)
  Tank1/1(LL1) -> LL1/1, Tank3/6(LL1)
  E3/1 -> Tank3/3(E3)
  F1/1 -> Tank1/2(F1)
  E1/1 -> Tank1/3(E1)
  CT3/1 -> Tank3/1(CT3)
  F3/1 -> Tank3/2(F3)
  EB3/1 -> Tank3/5(EB3)
  T3/1 -> Tank3/4(T3)
  CT1/1 -> Tank1/1(CT1)

== system c00005M_harness/M028 ==
  note: VALUES
      | ---------------------------------
      | ControlType = 1 | 2 | 3
      | FillTank = 0 | 1
      | EmptyTank = 0 | 1
      | ManualReference between 0 and 1
      | Tempreature between 0 and 100
      | EmergencyButton = 0 | 1
      | LiquidLevel between 0 and 1 (hmax)
  note: Inputs For Tank2
  note: NAMES
      | --------------------------------------------
      | CT1 = ControlType Tank 1
      | F1 = Fill Tank 1
      | E1 = Empty Tank 1
      | MR1 = Manual Reference Tank1
      | T1 = Temperature Tank 1
      | EB1 = Emergency Button Tank 1
      | LL1 = Liquid Level 1
  note: Inputs For Tank3
  note: Inputs For Tank1
  CT1 : Inport
  F1 : Inport  Port=2
  E1 : Inport  Port=3
  T1 : Inport  Port=4
  EB1 : Inport  Port=5
  CT3 : Inport  Port=6
  F3 : Inport  Port=7
  E3 : Inport  Port=8
  T3 : Inport  Port=9
  EB3 : Inport  Port=10
  Tank1 : Subsystem
  Tank3 : Subsystem
  LL1 : Outport
  LL3 : Outport  Port=2
  wires:
  EB1/1 -> Tank1/5(EB1)
  Tank3/1(LL3) -> LL3/1, Tank1/6(LL3)
  T1/1 -> Tank1/4(T1)
  Tank1/1(LL1) -> LL1/1, Tank3/6(LL1)
  E3/1 -> Tank3/3(E3)
  F1/1 -> Tank1/2(F1)
  E1/1 -> Tank1/3(E1)
  CT3/1 -> Tank3/1(CT3)
  F3/1 -> Tank3/2(F3)
  EB3/1 -> Tank3/5(EB3)
  T3/1 -> Tank3/4(T3)
  CT1/1 -> Tank1/1(CT1)

== system c00005M_harness/M029 ==
  note: VALUES
      | ---------------------------------
      | ControlType = 1 | 2 | 3
      | FillTank = 0 | 1
      | EmptyTank = 0 | 1
      | ManualReference between 0 and 1
      | Tempreature between 0 and 100
      | EmergencyButton = 0 | 1
      | LiquidLevel between 0 and 1 (hmax)
  note: Inputs For Tank2
  note: NAMES
      | --------------------------------------------
      | CT1 = ControlType Tank 1
      | F1 = Fill Tank 1
      | E1 = Empty Tank 1
      | MR1 = Manual Reference Tank1
      | T1 = Temperature Tank 1
      | EB1 = Emergency Button Tank 1
      | LL1 = Liquid Level 1
  note: Inputs For Tank3
  note: Inputs For Tank1
  CT1 : Inport
  F1 : Inport  Port=2
  E1 : Inport  Port=3
  T1 : Inport  Port=4
  EB1 : Inport  Port=5
  CT3 : Inport  Port=6
  F3 : Inport  Port=7
  E3 : Inport  Port=8
  T3 : Inport  Port=9
  EB3 : Inport  Port=10
  Tank1 : Subsystem
  Tank3 : Subsystem
  LL1 : Outport
  LL3 : Outport  Port=2
  wires:
  EB1/1 -> Tank1/5(EB1)
  Tank3/1(LL3) -> LL3/1, Tank1/6(LL3)
  T1/1 -> Tank1/4(T1)
  Tank1/1(LL1) -> LL1/1, Tank3/6(LL1)
  E3/1 -> Tank3/3(E3)
  F1/1 -> Tank1/2(F1)
  E1/1 -> Tank1/3(E1)
  CT3/1 -> Tank3/1(CT3)
  F3/1 -> Tank3/2(F3)
  EB3/1 -> Tank3/5(EB3)
  T3/1 -> Tank3/4(T3)
  CT1/1 -> Tank1/1(CT1)

== system c00005M_harness/M030 ==
  note: VALUES
      | ---------------------------------
      | ControlType = 1 | 2 | 3
      | FillTank = 0 | 1
      | EmptyTank = 0 | 1
      | ManualReference between 0 and 1
      | Tempreature between 0 and 100
      | EmergencyButton = 0 | 1
      | LiquidLevel between 0 and 1 (hmax)
  note: Inputs For Tank2
  note: NAMES
      | --------------------------------------------
      | CT1 = ControlType Tank 1
      | F1 = Fill Tank 1
      | E1 = Empty Tank 1
      | MR1 = Manual Reference Tank1
      | T1 = Temperature Tank 1
      | EB1 = Emergency Button Tank 1
      | LL1 = Liquid Level 1
  note: Inputs For Tank3
  note: Inputs For Tank1
  CT1 : Inport
  F1 : Inport  Port=2
  E1 : Inport  Port=3
  T1 : Inport  Port=4
  EB1 : Inport  Port=5
  CT3 : Inport  Port=6
  F3 : Inport  Port=7
  E3 : Inport  Port=8
  T3 : Inport  Port=9
  EB3 : Inport  Port=10
  Tank1 : Subsystem
  Tank3 : Subsystem
  LL1 : Outport
  LL3 : Outport  Port=2
  wires:
  EB1/1 -> Tank1/5(EB1)
  Tank3/1(LL3) -> LL3/1, Tank1/6(LL3)
  T1/1 -> Tank1/4(T1)
  Tank1/1(LL1) -> LL1/1, Tank3/6(LL1)
  E3/1 -> Tank3/3(E3)
  F1/1 -> Tank1/2(F1)
  E1/1 -> Tank1/3(E1)
  CT3/1 -> Tank3/1(CT3)
  F3/1 -> Tank3/2(F3)
  EB3/1 -> Tank3/5(EB3)
  T3/1 -> Tank3/4(T3)
  CT1/1 -> Tank1/1(CT1)

== system c00005M_harness/M031 ==
  note: VALUES
      | ---------------------------------
      | ControlType = 1 | 2 | 3
      | FillTank = 0 | 1
      | EmptyTank = 0 | 1
      | ManualReference between 0 and 1
      | Tempreature between 0 and 100
      | EmergencyButton = 0 | 1
      | LiquidLevel between 0 and 1 (hmax)
  note: Inputs For Tank2
  note: NAMES
      | --------------------------------------------
      | CT1 = ControlType Tank 1
      | F1 = Fill Tank 1
      | E1 = Empty Tank 1
      | MR1 = Manual Reference Tank1
      | T1 = Temperature Tank 1
      | EB1 = Emergency Button Tank 1
      | LL1 = Liquid Level 1
  note: Inputs For Tank3
  note: Inputs For Tank1
  CT1 : Inport
  F1 : Inport  Port=2
  E1 : Inport  Port=3
  T1 : Inport  Port=4
  EB1 : Inport  Port=5
  CT3 : Inport  Port=6
  F3 : Inport  Port=7
  E3 : Inport  Port=8
  T3 : Inport  Port=9
  EB3 : Inport  Port=10
  Tank1 : Subsystem
  Tank3 : Subsystem
  LL1 : Outport
  LL3 : Outport  Port=2
  wires:
  EB1/1 -> Tank1/5(EB1)
  Tank3/1(LL3) -> LL3/1, Tank1/6(LL3)
  T1/1 -> Tank1/4(T1)
  Tank1/1(LL1) -> LL1/1, Tank3/6(LL1)
  E3/1 -> Tank3/3(E3)
  F1/1 -> Tank1/2(F1)
  E1/1 -> Tank1/3(E1)
  CT3/1 -> Tank3/1(CT3)
  F3/1 -> Tank3/2(F3)
  EB3/1 -> Tank3/5(EB3)
  T3/1 -> Tank3/4(T3)
  CT1/1 -> Tank1/1(CT1)

== system c00005M_harness/M032 ==
  note: VALUES
      | ---------------------------------
      | ControlType = 1 | 2 | 3
      | FillTank = 0 | 1
      | EmptyTank = 0 | 1
      | ManualReference between 0 and 1
      | Tempreature between 0 and 100
      | EmergencyButton = 0 | 1
      | LiquidLevel between 0 and 1 (hmax)
  note: Inputs For Tank2
  note: NAMES
      | --------------------------------------------
      | CT1 = ControlType Tank 1
      | F1 = Fill Tank 1
      | E1 = Empty Tank 1
      | MR1 = Manual Reference Tank1
      | T1 = Temperature Tank 1
      | EB1 = Emergency Button Tank 1
      | LL1 = Liquid Level 1
  note: Inputs For Tank3
  note: Inputs For Tank1
  CT1 : Inport
  F1 : Inport  Port=2
  E1 : Inport  Port=3
  T1 : Inport  Port=4
  EB1 : Inport  Port=5
  CT3 : Inport  Port=6
  F3 : Inport  Port=7
  E3 : Inport  Port=8
  T3 : Inport  Port=9
  EB3 : Inport  Port=10
  Tank1 : Subsystem
  Tank3 : Subsystem
  LL1 : Outport
  LL3 : Outport  Port=2
  wires:
  EB1/1 -> Tank1/5(EB1)
  Tank3/1(LL3) -> LL3/1, Tank1/6(LL3)
  T1/1 -> Tank1/4(T1)
  Tank1/1(LL1) -> LL1/1, Tank3/6(LL1)
  E3/1 -> Tank3/3(E3)
  F1/1 -> Tank1/2(F1)
  E1/1 -> Tank1/3(E1)
  CT3/1 -> Tank3/1(CT3)
  F3/1 -> Tank3/2(F3)
  EB3/1 -> Tank3/5(EB3)
  T3/1 -> Tank3/4(T3)
  CT1/1 -> Tank1/1(CT1)

== system c00005M_harness/M033 ==
  note: VALUES
      | ---------------------------------
      | ControlType = 1 | 2 | 3
      | FillTank = 0 | 1
      | EmptyTank = 0 | 1
      | ManualReference between 0 and 1
      | Tempreature between 0 and 100
      | EmergencyButton = 0 | 1
      | LiquidLevel between 0 and 1 (hmax)
  note: Inputs For Tank2
  note: NAMES
      | --------------------------------------------
      | CT1 = ControlType Tank 1
      | F1 = Fill Tank 1
      | E1 = Empty Tank 1
      | MR1 = Manual Reference Tank1
      | T1 = Temperature Tank 1
      | EB1 = Emergency Button Tank 1
      | LL1 = Liquid Level 1
  note: Inputs For Tank3
  note: Inputs For Tank1
  CT1 : Inport
  F1 : Inport  Port=2
  E1 : Inport  Port=3
  T1 : Inport  Port=4
  EB1 : Inport  Port=5
  CT3 : Inport  Port=6
  F3 : Inport  Port=7
  E3 : Inport  Port=8
  T3 : Inport  Port=9
  EB3 : Inport  Port=10
  Tank1 : Subsystem
  Tank3 : Subsystem
  LL1 : Outport
  LL3 : Outport  Port=2
  wires:
  EB1/1 -> Tank1/5(EB1)
  Tank3/1(LL3) -> LL3/1, Tank1/6(LL3)
  T1/1 -> Tank1/4(T1)
  Tank1/1(LL1) -> LL1/1, Tank3/6(LL1)
  E3/1 -> Tank3/3(E3)
  F1/1 -> Tank1/2(F1)
  E1/1 -> Tank1/3(E1)
  CT3/1 -> Tank3/1(CT3)
  F3/1 -> Tank3/2(F3)
  EB3/1 -> Tank3/5(EB3)
  T3/1 -> Tank3/4(T3)
  CT1/1 -> Tank1/1(CT1)

== system c00005M_harness/M034 ==
  note: VALUES
      | ---------------------------------
      | ControlType = 1 | 2 | 3
      | FillTank = 0 | 1
      | EmptyTank = 0 | 1
      | ManualReference between 0 and 1
      | Tempreature between 0 and 100
      | EmergencyButton = 0 | 1
      | LiquidLevel between 0 and 1 (hmax)
  note: Inputs For Tank2
  note: NAMES
      | --------------------------------------------
      | CT1 = ControlType Tank 1
      | F1 = Fill Tank 1
      | E1 = Empty Tank 1
      | MR1 = Manual Reference Tank1
      | T1 = Temperature Tank 1
      | EB1 = Emergency Button Tank 1
      | LL1 = Liquid Level 1
  note: Inputs For Tank3
  note: Inputs For Tank1
  CT1 : Inport
  F1 : Inport  Port=2
  E1 : Inport  Port=3
  T1 : Inport  Port=4
  EB1 : Inport  Port=5
  CT3 : Inport  Port=6
  F3 : Inport  Port=7
  E3 : Inport  Port=8
  T3 : Inport  Port=9
  EB3 : Inport  Port=10
  Tank1 : Subsystem
  Tank3 : Subsystem
  LL1 : Outport
  LL3 : Outport  Port=2
  wires:
  EB1/1 -> Tank1/5(EB1)
  Tank3/1(LL3) -> LL3/1, Tank1/6(LL3)
  T1/1 -> Tank1/4(T1)
  Tank1/1(LL1) -> LL1/1, Tank3/6(LL1)
  E3/1 -> Tank3/3(E3)
  F1/1 -> Tank1/2(F1)
  E1/1 -> Tank1/3(E1)
  CT3/1 -> Tank3/1(CT3)
  F3/1 -> Tank3/2(F3)
  EB3/1 -> Tank3/5(EB3)
  T3/1 -> Tank3/4(T3)
  CT1/1 -> Tank1/1(CT1)

== system c00005M_harness/M035 ==
  note: VALUES
      | ---------------------------------
      | ControlType = 1 | 2 | 3
      | FillTank = 0 | 1
      | EmptyTank = 0 | 1
      | ManualReference between 0 and 1
      | Tempreature between 0 and 100
      | EmergencyButton = 0 | 1
      | LiquidLevel between 0 and 1 (hmax)
  note: Inputs For Tank2
  note: NAMES
      | --------------------------------------------
      | CT1 = ControlType Tank 1
      | F1 = Fill Tank 1
      | E1 = Empty Tank 1
      | MR1 = Manual Reference Tank1
      | T1 = Temperature Tank 1
      | EB1 = Emergency Button Tank 1
      | LL1 = Liquid Level 1
  note: Inputs For Tank3
  note: Inputs For Tank1
  CT1 : Inport
  F1 : Inport  Port=2
  E1 : Inport  Port=3
  T1 : Inport  Port=4
  EB1 : Inport  Port=5
  CT3 : Inport  Port=6
  F3 : Inport  Port=7
  E3 : Inport  Port=8
  T3 : Inport  Port=9
  EB3 : Inport  Port=10
  Tank1 : Subsystem
  Tank3 : Subsystem
  LL1 : Outport
  LL3 : Outport  Port=2
  wires:
  EB1/1 -> Tank1/5(EB1)
  Tank3/1(LL3) -> LL3/1, Tank1/6(LL3)
  T1/1 -> Tank1/4(T1)
  Tank1/1(LL1) -> LL1/1, Tank3/6(LL1)
  E3/1 -> Tank3/3(E3)
  F1/1 -> Tank1/2(F1)
  E1/1 -> Tank1/3(E1)
  CT3/1 -> Tank3/1(CT3)
  F3/1 -> Tank3/2(F3)
  EB3/1 -> Tank3/5(EB3)
  T3/1 -> Tank3/4(T3)
  CT1/1 -> Tank1/1(CT1)

== system c00005M_harness/M036 ==
  note: VALUES
      | ---------------------------------
      | ControlType = 1 | 2 | 3
      | FillTank = 0 | 1
      | EmptyTank = 0 | 1
      | ManualReference between 0 and 1
      | Tempreature between 0 and 100
      | EmergencyButton = 0 | 1
      | LiquidLevel between 0 and 1 (hmax)
  note: Inputs For Tank2
  note: NAMES
      | --------------------------------------------
      | CT1 = ControlType Tank 1
      | F1 = Fill Tank 1
      | E1 = Empty Tank 1
      | MR1 = Manual Reference Tank1
      | T1 = Temperature Tank 1
      | EB1 = Emergency Button Tank 1
      | LL1 = Liquid Level 1
  note: Inputs For Tank3
  note: Inputs For Tank1
  CT1 : Inport
  F1 : Inport  Port=2
  E1 : Inport  Port=3
  T1 : Inport  Port=4
  EB1 : Inport  Port=5
  CT3 : Inport  Port=6
  F3 : Inport  Port=7
  E3 : Inport  Port=8
  T3 : Inport  Port=9
  EB3 : Inport  Port=10
  Tank1 : Subsystem
  Tank3 : Subsystem
  LL1 : Outport
  LL3 : Outport  Port=2
  wires:
  EB1/1 -> Tank1/5(EB1)
  Tank3/1(LL3) -> LL3/1, Tank1/6(LL3)
  T1/1 -> Tank1/4(T1)
  Tank1/1(LL1) -> LL1/1, Tank3/6(LL1)
  E3/1 -> Tank3/3(E3)
  F1/1 -> Tank1/2(F1)
  E1/1 -> Tank1/3(E1)
  CT3/1 -> Tank3/1(CT3)
  F3/1 -> Tank3/2(F3)
  EB3/1 -> Tank3/5(EB3)
  T3/1 -> Tank3/4(T3)
  CT1/1 -> Tank1/1(CT1)

== system c00005M_harness/M037 ==
  note: VALUES
      | ---------------------------------
      | ControlType = 1 | 2 | 3
      | FillTank = 0 | 1
      | EmptyTank = 0 | 1
      | ManualReference between 0 and 1
      | Tempreature between 0 and 100
      | EmergencyButton = 0 | 1
      | LiquidLevel between 0 and 1 (hmax)
  note: Inputs For Tank2
  note: NAMES
      | --------------------------------------------
      | CT1 = ControlType Tank 1
      | F1 = Fill Tank 1
      | E1 = Empty Tank 1
      | MR1 = Manual Reference Tank1
      | T1 = Temperature Tank 1
      | EB1 = Emergency Button Tank 1
      | LL1 = Liquid Level 1
  note: Inputs For Tank3
  note: Inputs For Tank1
  CT1 : Inport
  F1 : Inport  Port=2
  E1 : Inport  Port=3
  T1 : Inport  Port=4
  EB1 : Inport  Port=5
  CT3 : Inport  Port=6
  F3 : Inport  Port=7
  E3 : Inport  Port=8
  T3 : Inport  Port=9
  EB3 : Inport  Port=10
  Tank1 : Subsystem
  Tank3 : Subsystem
  LL1 : Outport
  LL3 : Outport  Port=2
  wires:
  EB1/1 -> Tank1/5(EB1)
  Tank3/1(LL3) -> LL3/1, Tank1/6(LL3)
  T1/1 -> Tank1/4(T1)
  Tank1/1(LL1) -> LL1/1, Tank3/6(LL1)
  E3/1 -> Tank3/3(E3)
  F1/1 -> Tank1/2(F1)
  E1/1 -> Tank1/3(E1)
  CT3/1 -> Tank3/1(CT3)
  F3/1 -> Tank3/2(F3)
  EB3/1 -> Tank3/5(EB3)
  T3/1 -> Tank3/4(T3)
  CT1/1 -> Tank1/1(CT1)

== system c00005M_harness/M038 ==
  note: VALUES
      | ---------------------------------
      | ControlType = 1 | 2 | 3
      | FillTank = 0 | 1
      | EmptyTank = 0 | 1
      | ManualReference between 0 and 1
      | Tempreature between 0 and 100
      | EmergencyButton = 0 | 1
      | LiquidLevel between 0 and 1 (hmax)
  note: Inputs For Tank2
  note: NAMES
      | --------------------------------------------
      | CT1 = ControlType Tank 1
      | F1 = Fill Tank 1
      | E1 = Empty Tank 1
      | MR1 = Manual Reference Tank1
      | T1 = Temperature Tank 1
      | EB1 = Emergency Button Tank 1
      | LL1 = Liquid Level 1
  note: Inputs For Tank3
  note: Inputs For Tank1
  CT1 : Inport
  F1 : Inport  Port=2
  E1 : Inport  Port=3
  T1 : Inport  Port=4
  EB1 : Inport  Port=5
  CT3 : Inport  Port=6
  F3 : Inport  Port=7
  E3 : Inport  Port=8
  T3 : Inport  Port=9
  EB3 : Inport  Port=10
  Tank1 : Subsystem
  Tank3 : Subsystem
  LL1 : Outport
  LL3 : Outport  Port=2
  wires:
  EB1/1 -> Tank1/5(EB1)
  Tank3/1(LL3) -> LL3/1, Tank1/6(LL3)
  T1/1 -> Tank1/4(T1)
  Tank1/1(LL1) -> LL1/1, Tank3/6(LL1)
  E3/1 -> Tank3/3(E3)
  F1/1 -> Tank1/2(F1)
  E1/1 -> Tank1/3(E1)
  CT3/1 -> Tank3/1(CT3)
  F3/1 -> Tank3/2(F3)
  EB3/1 -> Tank3/5(EB3)
  T3/1 -> Tank3/4(T3)
  CT1/1 -> Tank1/1(CT1)

== system c00005M_harness/M039 ==
  note: VALUES
      | ---------------------------------
      | ControlType = 1 | 2 | 3
      | FillTank = 0 | 1
      | EmptyTank = 0 | 1
      | ManualReference between 0 and 1
      | Tempreature between 0 and 100
      | EmergencyButton = 0 | 1
      | LiquidLevel between 0 and 1 (hmax)
  note: Inputs For Tank2
  note: NAMES
      | --------------------------------------------
      | CT1 = ControlType Tank 1
      | F1 = Fill Tank 1
      | E1 = Empty Tank 1
      | MR1 = Manual Reference Tank1
      | T1 = Temperature Tank 1
      | EB1 = Emergency Button Tank 1
      | LL1 = Liquid Level 1
  note: Inputs For Tank3
  note: Inputs For Tank1
  CT1 : Inport
  F1 : Inport  Port=2
  E1 : Inport  Port=3
  T1 : Inport  Port=4
  EB1 : Inport  Port=5
  CT3 : Inport  Port=6
  F3 : Inport  Port=7
  E3 : Inport  Port=8
  T3 : Inport  Port=9
  EB3 : Inport  Port=10
  Tank1 : Subsystem
  Tank3 : Subsystem
  LL1 : Outport
  LL3 : Outport  Port=2
  wires:
  EB1/1 -> Tank1/5(EB1)
  Tank3/1(LL3) -> LL3/1, Tank1/6(LL3)
  T1/1 -> Tank1/4(T1)
  Tank1/1(LL1) -> LL1/1, Tank3/6(LL1)
  E3/1 -> Tank3/3(E3)
  F1/1 -> Tank1/2(F1)
  E1/1 -> Tank1/3(E1)
  CT3/1 -> Tank3/1(CT3)
  F3/1 -> Tank3/2(F3)
  EB3/1 -> Tank3/5(EB3)
  T3/1 -> Tank3/4(T3)
  CT1/1 -> Tank1/1(CT1)

== system c00005M_harness/M040 ==
  note: VALUES
      | ---------------------------------
      | ControlType = 1 | 2 | 3
      | FillTank = 0 | 1
      | EmptyTank = 0 | 1
      | ManualReference between 0 and 1
      | Tempreature between 0 and 100
      | EmergencyButton = 0 | 1
      | LiquidLevel between 0 and 1 (hmax)
  note: Inputs For Tank2
  note: NAMES
      | --------------------------------------------
      | CT1 = ControlType Tank 1
      | F1 = Fill Tank 1
      | E1 = Empty Tank 1
      | MR1 = Manual Reference Tank1
      | T1 = Temperature Tank 1
      | EB1 = Emergency Button Tank 1
      | LL1 = Liquid Level 1
  note: Inputs For Tank3
  note: Inputs For Tank1
  CT1 : Inport
  F1 : Inport  Port=2
  E1 : Inport  Port=3
  T1 : Inport  Port=4
  EB1 : Inport  Port=5
  CT3 : Inport  Port=6
  F3 : Inport  Port=7
  E3 : Inport  Port=8
  T3 : Inport  Port=9
  EB3 : Inport  Port=10
  Tank1 : Subsystem
  Tank3 : Subsystem
  LL1 : Outport
  LL3 : Outport  Port=2
  wires:
  EB1/1 -> Tank1/5(EB1)
  Tank3/1(LL3) -> LL3/1, Tank1/6(LL3)
  T1/1 -> Tank1/4(T1)
  Tank1/1(LL1) -> LL1/1, Tank3/6(LL1)
  E3/1 -> Tank3/3(E3)
  F1/1 -> Tank1/2(F1)
  E1/1 -> Tank1/3(E1)
  CT3/1 -> Tank3/1(CT3)
  F3/1 -> Tank3/2(F3)
  EB3/1 -> Tank3/5(EB3)
  T3/1 -> Tank3/4(T3)
  CT1/1 -> Tank1/1(CT1)

== system c00005M_harness/M041 ==
  note: VALUES
      | ---------------------------------
      | ControlType = 1 | 2 | 3
      | FillTank = 0 | 1
      | EmptyTank = 0 | 1
      | ManualReference between 0 and 1
      | Tempreature between 0 and 100
      | EmergencyButton = 0 | 1
      | LiquidLevel between 0 and 1 (hmax)
  note: Inputs For Tank2
  note: NAMES
      | --------------------------------------------
      | CT1 = ControlType Tank 1
      | F1 = Fill Tank 1
      | E1 = Empty Tank 1
      | MR1 = Manual Reference Tank1
      | T1 = Temperature Tank 1
      | EB1 = Emergency Button Tank 1
      | LL1 = Liquid Level 1
  note: Inputs For Tank3
  note: Inputs For Tank1
  CT1 : Inport
  F1 : Inport  Port=2
  E1 : Inport  Port=3
  T1 : Inport  Port=4
  EB1 : Inport  Port=5
  CT3 : Inport  Port=6
  F3 : Inport  Port=7
  E3 : Inport  Port=8
  T3 : Inport  Port=9
  EB3 : Inport  Port=10
  Tank1 : Subsystem
  Tank3 : Subsystem
  LL1 : Outport
  LL3 : Outport  Port=2
  wires:
  EB1/1 -> Tank1/5(EB1)
  Tank3/1(LL3) -> LL3/1, Tank1/6(LL3)
  T1/1 -> Tank1/4(T1)
  Tank1/1(LL1) -> LL1/1, Tank3/6(LL1)
  E3/1 -> Tank3/3(E3)
  F1/1 -> Tank1/2(F1)
  E1/1 -> Tank1/3(E1)
  CT3/1 -> Tank3/1(CT3)
  F3/1 -> Tank3/2(F3)
  EB3/1 -> Tank3/5(EB3)
  T3/1 -> Tank3/4(T3)
  CT1/1 -> Tank1/1(CT1)

== system c00005M_harness/M042 ==
  note: VALUES
      | ---------------------------------
      | ControlType = 1 | 2 | 3
      | FillTank = 0 | 1
      | EmptyTank = 0 | 1
      | ManualReference between 0 and 1
      | Tempreature between 0 and 100
      | EmergencyButton = 0 | 1
      | LiquidLevel between 0 and 1 (hmax)
  note: Inputs For Tank2
  note: NAMES
      | --------------------------------------------
      | CT1 = ControlType Tank 1
      | F1 = Fill Tank 1
      | E1 = Empty Tank 1
      | MR1 = Manual Reference Tank1
      | T1 = Temperature Tank 1
      | EB1 = Emergency Button Tank 1
      | LL1 = Liquid Level 1
  note: Inputs For Tank3
  note: Inputs For Tank1
  CT1 : Inport
  F1 : Inport  Port=2
  E1 : Inport  Port=3
  T1 : Inport  Port=4
  EB1 : Inport  Port=5
  CT3 : Inport  Port=6
  F3 : Inport  Port=7
  E3 : Inport  Port=8
  T3 : Inport  Port=9
  EB3 : Inport  Port=10
  Tank1 : Subsystem
  Tank3 : Subsystem
  LL1 : Outport
  LL3 : Outport  Port=2
  wires:
  EB1/1 -> Tank1/5(EB1)
  Tank3/1(LL3) -> LL3/1, Tank1/6(LL3)
  T1/1 -> Tank1/4(T1)
  Tank1/1(LL1) -> LL1/1, Tank3/6(LL1)
  E3/1 -> Tank3/3(E3)
  F1/1 -> Tank1/2(F1)
  E1/1 -> Tank1/3(E1)
  CT3/1 -> Tank3/1(CT3)
  F3/1 -> Tank3/2(F3)
  EB3/1 -> Tank3/5(EB3)
  T3/1 -> Tank3/4(T3)
  CT1/1 -> Tank1/1(CT1)

== system c00005M_harness/M043 ==
  note: VALUES
      | ---------------------------------
      | ControlType = 1 | 2 | 3
      | FillTank = 0 | 1
      | EmptyTank = 0 | 1
      | ManualReference between 0 and 1
      | Tempreature between 0 and 100
      | EmergencyButton = 0 | 1
      | LiquidLevel between 0 and 1 (hmax)
  note: Inputs For Tank2
  note: NAMES
      | --------------------------------------------
      | CT1 = ControlType Tank 1
      | F1 = Fill Tank 1
      | E1 = Empty Tank 1
      | MR1 = Manual Reference Tank1
      | T1 = Temperature Tank 1
      | EB1 = Emergency Button Tank 1
      | LL1 = Liquid Level 1
  note: Inputs For Tank3
  note: Inputs For Tank1
  CT1 : Inport
  F1 : Inport  Port=2
  E1 : Inport  Port=3
  T1 : Inport  Port=4
  EB1 : Inport  Port=5
  CT3 : Inport  Port=6
  F3 : Inport  Port=7
  E3 : Inport  Port=8
  T3 : Inport  Port=9
  EB3 : Inport  Port=10
  Tank1 : Subsystem
  Tank3 : Subsystem
  LL1 : Outport
  LL3 : Outport  Port=2
  wires:
  EB1/1 -> Tank1/5(EB1)
  Tank3/1(LL3) -> LL3/1, Tank1/6(LL3)
  T1/1 -> Tank1/4(T1)
  Tank1/1(LL1) -> LL1/1, Tank3/6(LL1)
  E3/1 -> Tank3/3(E3)
  F1/1 -> Tank1/2(F1)
  E1/1 -> Tank1/3(E1)
  CT3/1 -> Tank3/1(CT3)
  F3/1 -> Tank3/2(F3)
  EB3/1 -> Tank3/5(EB3)
  T3/1 -> Tank3/4(T3)
  CT1/1 -> Tank1/1(CT1)

== system c00005M_harness/M044 ==
  note: VALUES
      | ---------------------------------
      | ControlType = 1 | 2 | 3
      | FillTank = 0 | 1
      | EmptyTank = 0 | 1
      | ManualReference between 0 and 1
      | Tempreature between 0 and 100
      | EmergencyButton = 0 | 1
      | LiquidLevel between 0 and 1 (hmax)
  note: Inputs For Tank2
  note: NAMES
      | --------------------------------------------
      | CT1 = ControlType Tank 1
      | F1 = Fill Tank 1
      | E1 = Empty Tank 1
      | MR1 = Manual Reference Tank1
      | T1 = Temperature Tank 1
      | EB1 = Emergency Button Tank 1
      | LL1 = Liquid Level 1
  note: Inputs For Tank3
  note: Inputs For Tank1
  CT1 : Inport
  F1 : Inport  Port=2
  E1 : Inport  Port=3
  T1 : Inport  Port=4
  EB1 : Inport  Port=5
  CT3 : Inport  Port=6
  F3 : Inport  Port=7
  E3 : Inport  Port=8
  T3 : Inport  Port=9
  EB3 : Inport  Port=10
  Tank1 : Subsystem
  Tank3 : Subsystem
  LL1 : Outport
  LL3 : Outport  Port=2
  wires:
  EB1/1 -> Tank1/5(EB1)
  Tank3/1(LL3) -> LL3/1, Tank1/6(LL3)
  T1/1 -> Tank1/4(T1)
  Tank1/1(LL1) -> LL1/1, Tank3/6(LL1)
  E3/1 -> Tank3/3(E3)
  F1/1 -> Tank1/2(F1)
  E1/1 -> Tank1/3(E1)
  CT3/1 -> Tank3/1(CT3)
  F3/1 -> Tank3/2(F3)
  EB3/1 -> Tank3/5(EB3)
  T3/1 -> Tank3/4(T3)
  CT1/1 -> Tank1/1(CT1)

== system c00005M_harness/M045 ==
  note: VALUES
      | ---------------------------------
      | ControlType = 1 | 2 | 3
      | FillTank = 0 | 1
      | EmptyTank = 0 | 1
      | ManualReference between 0 and 1
      | Tempreature between 0 and 100
      | EmergencyButton = 0 | 1
      | LiquidLevel between 0 and 1 (hmax)
  note: Inputs For Tank2
  note: NAMES
      | --------------------------------------------
      | CT1 = ControlType Tank 1
      | F1 = Fill Tank 1
      | E1 = Empty Tank 1
      | MR1 = Manual Reference Tank1
      | T1 = Temperature Tank 1
      | EB1 = Emergency Button Tank 1
      | LL1 = Liquid Level 1
  note: Inputs For Tank3
  note: Inputs For Tank1
  CT1 : Inport
  F1 : Inport  Port=2
  E1 : Inport  Port=3
  T1 : Inport  Port=4
  EB1 : Inport  Port=5
  CT3 : Inport  Port=6
  F3 : Inport  Port=7
  E3 : Inport  Port=8
  T3 : Inport  Port=9
  EB3 : Inport  Port=10
  Tank1 : Subsystem
  Tank3 : Subsystem
  LL1 : Outport
  LL3 : Outport  Port=2
  wires:
  EB1/1 -> Tank1/5(EB1)
  Tank3/1(LL3) -> LL3/1, Tank1/6(LL3)
  T1/1 -> Tank1/4(T1)
  Tank1/1(LL1) -> LL1/1, Tank3/6(LL1)
  E3/1 -> Tank3/3(E3)
  F1/1 -> Tank1/2(F1)
  E1/1 -> Tank1/3(E1)
  CT3/1 -> Tank3/1(CT3)
  F3/1 -> Tank3/2(F3)
  EB3/1 -> Tank3/5(EB3)
  T3/1 -> Tank3/4(T3)
  CT1/1 -> Tank1/1(CT1)

== system c00005M_harness/M057 ==
  note: VALUES
      | ---------------------------------
      | ControlType = 1 | 2 | 3
      | FillTank = 0 | 1
      | EmptyTank = 0 | 1
      | ManualReference between 0 and 1
      | Tempreature between 0 and 100
      | EmergencyButton = 0 | 1
      | LiquidLevel between 0 and 1 (hmax)
  note: Inputs For Tank2
  note: NAMES
      | --------------------------------------------
      | CT1 = ControlType Tank 1
      | F1 = Fill Tank 1
      | E1 = Empty Tank 1
      | MR1 = Manual Reference Tank1
      | T1 = Temperature Tank 1
      | EB1 = Emergency Button Tank 1
      | LL1 = Liquid Level 1
  note: Inputs For Tank3
  note: Inputs For Tank1
  CT1 : Inport
  F1 : Inport  Port=2
  E1 : Inport  Port=3
  T1 : Inport  Port=4
  EB1 : Inport  Port=5
  CT3 : Inport  Port=6
  F3 : Inport  Port=7
  E3 : Inport  Port=8
  T3 : Inport  Port=9
  EB3 : Inport  Port=10
  Tank1 : Subsystem
  Tank3 : Subsystem
  LL1 : Outport
  LL3 : Outport  Port=2
  wires:
  EB1/1 -> Tank1/5(EB1)
  Tank3/1(LL3) -> LL3/1, Tank1/6(LL3)
  T1/1 -> Tank1/4(T1)
  Tank1/1(LL1) -> LL1/1, Tank3/6(LL1)
  E3/1 -> Tank3/3(E3)
  F1/1 -> Tank1/2(F1)
  E1/1 -> Tank1/3(E1)
  CT3/1 -> Tank3/1(CT3)
  F3/1 -> Tank3/2(F3)
  EB3/1 -> Tank3/5(EB3)
  T3/1 -> Tank3/4(T3)
  CT1/1 -> Tank1/1(CT1)

== system c00005M_harness/M058 ==
  note: VALUES
      | ---------------------------------
      | ControlType = 1 | 2 | 3
      | FillTank = 0 | 1
      | EmptyTank = 0 | 1
      | ManualReference between 0 and 1
      | Tempreature between 0 and 100
      | EmergencyButton = 0 | 1
      | LiquidLevel between 0 and 1 (hmax)
  note: Inputs For Tank2
  note: NAMES
      | --------------------------------------------
      | CT1 = ControlType Tank 1
      | F1 = Fill Tank 1
      | E1 = Empty Tank 1
      | MR1 = Manual Reference Tank1
      | T1 = Temperature Tank 1
      | EB1 = Emergency Button Tank 1
      | LL1 = Liquid Level 1
  note: Inputs For Tank3
  note: Inputs For Tank1
  CT1 : Inport
  F1 : Inport  Port=2
  E1 : Inport  Port=3
  T1 : Inport  Port=4
  EB1 : Inport  Port=5
  CT3 : Inport  Port=6
  F3 : Inport  Port=7
  E3 : Inport  Port=8
  T3 : Inport  Port=9
  EB3 : Inport  Port=10
  Tank1 : Subsystem
  Tank3 : Subsystem
  LL1 : Outport
  LL3 : Outport  Port=2
  wires:
  EB1/1 -> Tank1/5(EB1)
  Tank3/1(LL3) -> LL3/1, Tank1/6(LL3)
  T1/1 -> Tank1/4(T1)
  Tank1/1(LL1) -> LL1/1, Tank3/6(LL1)
  E3/1 -> Tank3/3(E3)
  F1/1 -> Tank1/2(F1)
  E1/1 -> Tank1/3(E1)
  CT3/1 -> Tank3/1(CT3)
  F3/1 -> Tank3/2(F3)
  EB3/1 -> Tank3/5(EB3)
  T3/1 -> Tank3/4(T3)
  CT1/1 -> Tank1/1(CT1)

== system c00005M_harness/M059 ==
  note: VALUES
      | ---------------------------------
      | ControlType = 1 | 2 | 3
      | FillTank = 0 | 1
      | EmptyTank = 0 | 1
      | ManualReference between 0 and 1
      | Tempreature between 0 and 100
      | EmergencyButton = 0 | 1
      | LiquidLevel between 0 and 1 (hmax)
  note: Inputs For Tank2
  note: NAMES
      | --------------------------------------------
      | CT1 = ControlType Tank 1
      | F1 = Fill Tank 1
      | E1 = Empty Tank 1
      | MR1 = Manual Reference Tank1
      | T1 = Temperature Tank 1
      | EB1 = Emergency Button Tank 1
      | LL1 = Liquid Level 1
  note: Inputs For Tank3
  note: Inputs For Tank1
  CT1 : Inport
  F1 : Inport  Port=2
  E1 : Inport  Port=3
  T1 : Inport  Port=4
  EB1 : Inport  Port=5
  CT3 : Inport  Port=6
  F3 : Inport  Port=7
  E3 : Inport  Port=8
  T3 : Inport  Port=9
  EB3 : Inport  Port=10
  Tank1 : Subsystem
  Tank3 : Subsystem
  LL1 : Outport
  LL3 : Outport  Port=2
  wires:
  EB1/1 -> Tank1/5(EB1)
  Tank3/1(LL3) -> LL3/1, Tank1/6(LL3)
  T1/1 -> Tank1/4(T1)
  Tank1/1(LL1) -> LL1/1, Tank3/6(LL1)
  E3/1 -> Tank3/3(E3)
  F1/1 -> Tank1/2(F1)
  E1/1 -> Tank1/3(E1)
  CT3/1 -> Tank3/1(CT3)
  F3/1 -> Tank3/2(F3)
  EB3/1 -> Tank3/5(EB3)
  T3/1 -> Tank3/4(T3)
  CT1/1 -> Tank1/1(CT1)
